simulink model "ep_5_1_1"  (R2023b)
settings: Solver=VariableStepAuto  StartTime=0.0  StopTime=10.0  RelTol=1e-3
settings Model: Creator=86186  LastModifiedBy=86186

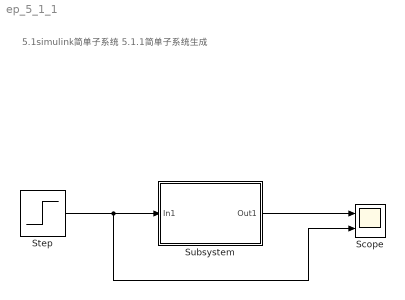
== system ep_5_1_1 ==
  note: 5.1simulink简单子系统
      | 5.1.1简单子系统生成
  Scope : Scope  NumInputPorts=2
  Step : Step  SampleTime=0
  Subsystem : Subsystem
  wires:
  Subsystem/1(Out1) -> Scope/1
  Step/1 -> Subsystem/1(In1), Scope/2

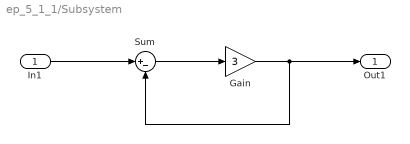
== system ep_5_1_1/Subsystem ==
  In1 : Inport
  Gain : Gain  Gain=3
  Sum : Sum  Inputs=|+-
  Out1 : Outport
  wires:
  In1/1 -> Sum/1
  Gain/1 -> Out1/1, Sum/2
  Sum/1 -> Gain/1
